simulink model "DynamicProprioTest"  (R2015a)
settings: Solver=ode4  SolverMode=MultiTasking  StartTime=0.0  StopTime=inf  FixedStep=BKIN_STEP_TIME  RelTol=1e-3
StartFcn:
  |  warndlg('Dexterit-E models cannot run under simulation. Please compile your model and run it from within Dexterit-E.');set_param(bdroot,'SimulationCommand','stop')
model workspace (MAT data in the model file):
  col_x = 1
  col_y = 2
  RADIUS_VIS = 3
  COLOR_INIT = 4
  BKIN_STEP_TIME = 0.00025
  START_WAIT_TIME_COL = 3
  E_END_TRIAL = 20
  STROKE_WIDTH = 6
  K_HAND_VEL = 1
  K_HOLDTIME = 2
  K_ROBOT_RAMP_TIME = 3
  E_ENABLED_CONTROLLER = 31
  K_TIME_TO_START = 4
  BKIN_KINEMATIC_FRAME_SIZE = 400
  E_NO_EVENT = 0
  ROTATION = 7
  E_WAIT_JS_THRESH = 16
  E_AT_JS_THRESH = 18
  STARTTARGET_COL = 1
  TIME_RETURNTOSTART_COL = 2
  MOVE_TIME_COL = 4
  TARGET_SHIFTTIME_COL = 5
  SHOWTARGETDUR_COL = 7
  MOVE_XVEL_COL = 9
  MOVE_YVEL_COL = 10
  E_INIT_TRIAL = 1
  E_MOVE_TO_START = 2
  E_AT_START = 4
  E_PASSIVE_HOLD_AT_START = 6
  E_MOVE_TO_END = 8
  COLOR_SELECT = 5
  ACTORPAS_COL = 11
  E_AT_END = 10
  DELAY_POSTTRIAL_COL = 8
  TARGETSHIFTDIR_COL = 6
  LABEL_HEIGHT = 8
  LABEL = 9
  E_ACTIVE_HOLD_AT_START = 7
  MVMT_VTHRESH_LB = 12
  MVMT_VTHRESH_UB = 13
  CHANNEL_WIDTH = 1
  WALL_WIDTH = 2
  WALL_STIFFNESS = 3
  WALL_VISCOSITY = 4
undefined symbols (not defined in the file): slselsubs
libraries: Video x6, simulink x5, slrtlib x5, General x3, KINARM_loads x3, KINARM_general x2, KINARM_IO x1, xpcnilib x1
(part 1 of 2)
CloseFcn:
  | rtwprivate ssgencode ModelCloseRequest b2lab2d
settings Model: ModifiedComment=chris -- Wed Feb 16 09:18:30 2005 -- Version 1.1384  ModifiedHistory=Feb 16/05 - Add error repeat, add offset ramp  ExtModeArmWhenConnect=off  ExtModeLogAll=off  Creator=Chris Grebeldinger  LastModifiedBy=User
settings SolverCC: EnableConcurrentExecution=on  AutoInsertRateTranBlk=on
settings DataIOCC: LimitDataPoints=off  SignalLoggingSaveFormat=ModelDataLogs  SaveOutput=off  SaveTime=off  SignalLoggingName=sigsOut
settings OptimizationCC: BlockReduction=off  BooleanDataType=off  OptimizeBlockIOStorage=off  BufferReuse=off  GlobalBufferReuse=off  ExpressionFolding=off  ExpressionDepthLimit=2147483647  LocalBlockOutputs=off  InitFltsAndDblsToZero=on
settings DebuggingCC: SaveWithParameterizedLinksMsg=none  UnderspecifiedInitializationDetection=Classic  MergeDetectMultiDrivingBlocksExec=none  SignalResolutionControl=TryResolveAllWithWarning  MultiTaskDSMMsg=warning  FcnCallInpInsideContextMsg=UseLocalSettings  StateNameClashWarn=warning  StrictBusMsg=ErrorOnBusTreatedAsVector
settings HardwareCC: ProdIntDivRoundTo=Zero  ProdEndianess=LittleEndian  ProdLongLongMode=on  ProdHWDeviceType=Generic->32-bit x86 compatible  TargetHWDeviceType=32-bit Generic
settings SFSimCC: SimCustomHeaderCode="#include \"stdlib.h\""  SFSimEcho=off  SimParseCustomCode=off
settings RTWCC: SystemTargetFile=slrt.tlc  TemplateMakefile=slrt_default_tmf  Description=Simulink Real-Time  CustomSourceCode="#include \"stdlib.h\""
settings CodeAppCC: MaxIdLength=63
settings SimulinkRealTimeCC: TargetFcnLib=ansi_tfl_tmw.mat  GeneratePreprocessorConditionals=Disable all  xPCisDownloadable=off  xPCisDefaultEnv=off

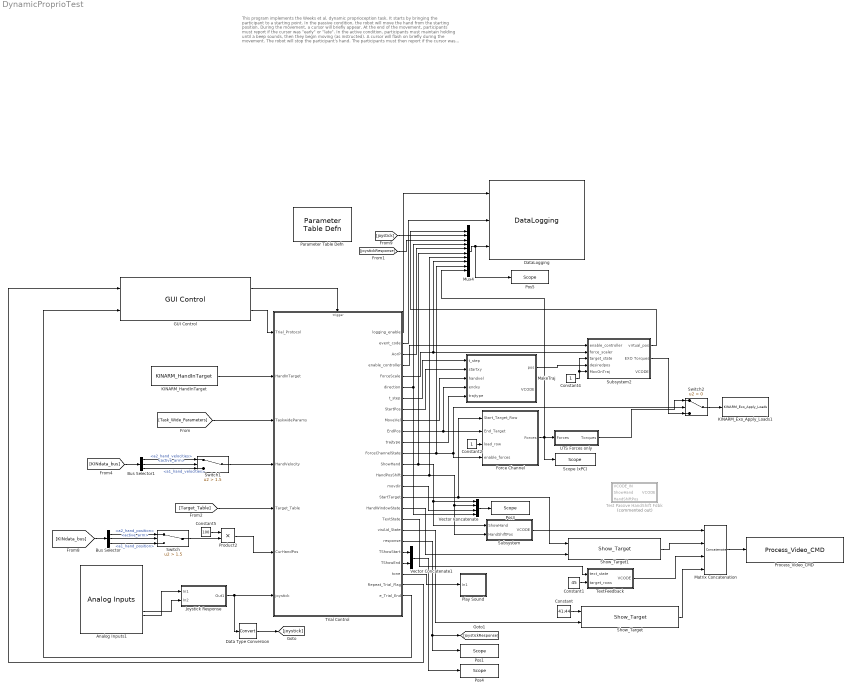
== system DynamicProprioTest ==
  note: This program implements the Weeks et al. dynamic proprioception task.
      | It starts by bringing the participant to a starting point.
      |
      | In the passive condition, the robot will move the hand from the starting position. During the movement, a cursor
      | will briefly appear. At the end of the movement, participants must report if the cursor was "early" or "late".
      |
      | In the active condition, participants must maintain holding
      | until a beep sounds, then they begin moving (as instructed). A cursor will flash on briefly during the movement.
      | The robot will stop the participant's hand. The participants must then report if the cursor was "early" or "late".
      | A force channel will enforce movement direction, and feedback will be used to adjust movement speed.
  Analog Inputs1 : KINARM_IO/Analog Inputs  channel=[1:32]  range=[5, 5, 5, 5, 5, 5, 5, 5,5, 5, 5, 5, 5, 5, 5, 5,5, 5, 5, 5, 5, 5, 5, 5,5, 5, 5, 5, 5, 5, 5, 5,]  coupling=[0, 0, 0, 0, 0, 0, 0, 0,0, 0, 0, 0, 0, 0, 0, 0,0, 0, 0, 0, 0, 0, 0, 0,0, 0, 0, 0, 0, 0, 0, 0,]  scantime6071e=1.28e-5  scantime6229=5e-6  sampletime=0.001  slot=-1  oscantime6071e=0
  Bus Selector : BusSelector  OutputSignals=Robot2.a2_hand_position,KINDataGeneral.active_arm,Robot1.a1_hand_position
  Bus Selector1 : BusSelector  OutputSignals=Robot2.a2_hand_velocities,KINDataGeneral.active_arm,Robot1.a1_hand_velocities
  Constant : Constant  Value=41:44
  Constant1 : Constant  Value=45
  Constant2 : Constant
  Constant4 : Constant
  Constant5 : Constant  Value=100
  Data Type Conversion : DataTypeConversion
  DataLogging : General/DataLogging  log_event_codes=on  log_analog_inputs=on  show_time_remaining=off
  Force Channel : Subsystem
  GUI Control : General/GUI Control  target_type_str=Circle  Target_Type=1  XYcols=[1 2]  Vcols=3  Lcols=4  indices_padding=[0 0 0 0;0 0 0 0]  task_version=1.0  show_repeat_trial_flag=on  target_table_rows=64  load_table_rows=20  tp_table_rows=100
  Joystick Response : Subsystem
  KINARM_Exo_Apply_Loads1 : KINARM_loads/KINARM_Exo_Apply_Loads  up_duration=200  down_duration=200  max_torque=12  limit_motors=off
  KINARM_HandInTarget : KINARM_general/KINARM_HandInTarget  use_dominant_hand=on  target_type=Rectangle  num_states=1  attribcol1=[RADIUS_VIS RADIUS_VIS 0]  attribcol2=[4 0 0]  attribcol3=[5 0 0]  attribcol4=[6 0 0]  attribcol5=[0 0 0]
  MakeTraj : Subsystem
  Matrix Concatenation : Concatenate  NumInputs=4  Mode=Multidimensional array
  Mux4 : Mux  Inputs=10
  Parameter Table Defn : General/Parameter Table Defn  ShowInLibBrowser=0
  Play Sound : Subsystem
  Pos1 : slrtlib/Displays and Logging/Scope   scopeno=2  scopetype=Target  autostart=on  viewmode=Numerical  formatstr='%15.6f'  grid=on  ylimits=[-10,10]  nosamples=250  noprepostsamples=0  interleave=1  triggermode=FreeRun  triggersignal=1  trigsignalfromport=off  triggerlevel=0.0  triggerslope=Either  triggerscope=1  triggersample=0  filename=data.dat  mode=Lazy  writesize=512  autorestart=off  dynamicfilemode=off  maxwritefilesize=512*1024^2
  Pos3 : slrtlib/Displays and Logging/Scope   scopeno=4  scopetype=Target  autostart=on  viewmode=Numerical  formatstr='%15.6f'  grid=on  ylimits=[-10,10]  nosamples=250  noprepostsamples=0  interleave=1  triggermode=FreeRun  triggersignal=1  trigsignalfromport=off  triggerlevel=0.0  triggerslope=Either  triggerscope=1  triggersample=0  filename=data.dat  mode=Lazy  writesize=512  autorestart=off  dynamicfilemode=off  maxwritefilesize=512*1024^2
  Pos4 : slrtlib/Displays and Logging/Scope   scopeno=5  scopetype=Target  autostart=on  viewmode=Numerical  formatstr='%15.6f'  grid=on  ylimits=[-10,10]  nosamples=250  noprepostsamples=0  interleave=1  triggermode=FreeRun  triggersignal=1  trigsignalfromport=off  triggerlevel=0.0  triggerslope=Either  triggerscope=1  triggersample=0  filename=data.dat  mode=Lazy  writesize=512  autorestart=off  dynamicfilemode=off  maxwritefilesize=512*1024^2
  Pos5 : slrtlib/Displays and Logging/Scope   scopeno=1  scopetype=Target  autostart=on  viewmode=Numerical  formatstr='%15.6f'  grid=on  ylimits=[-10,10]  nosamples=250  noprepostsamples=0  interleave=1  triggermode=FreeRun  triggersignal=1  trigsignalfromport=off  triggerlevel=0.0  triggerslope=Either  triggerscope=1  triggersample=0  filename=data.dat  mode=Lazy  writesize=512  autorestart=off  dynamicfilemode=off  maxwritefilesize=512*1024^2
  Process_Video_CMD : Video/Process_Video_CMD  video_delay=50
  Product2 : Product
  "Scope (xPC) " : slrtlib/Displays and Logging/Scope   scopeno=6  scopetype=Target  autostart=on  viewmode=Numerical  formatstr='%15.6f'  grid=on  ylimits=[0,0]  nosamples=250  noprepostsamples=0  interleave=1  triggermode=FreeRun  triggersignal=1  trigsignalfromport=off  triggerlevel=0.0  triggerslope=Either  triggerscope=1  triggersample=0  filename=data.dat  mode=Lazy  writesize=512  autorestart=off  dynamicfilemode=off  maxwritefilesize=512*1024^2
  Show_Target : Video/Show_Target  target_type=Triangle  num_states=2  attribcol1=[COLOR_INIT 0 0 RADIUS_VIS 0 0 ROTATION]  attribcol2=[COLOR_SELECT 0 0 RADIUS_VIS 0 0 ROTATION]  attribcol3=[0 0 0 0 0 0 0]  attribcol4=[0 0 0 0 0 0 0]  attribcol5=[0 0 24 0 0 0 0]  stateindices_padding=[0 0 0 0;0 0 0 0;0 0 0 0;0 0 0 0;0 0 0 0]  source=dialog  opacity=100  target_display=Both subject and operator displays  num_col=7
  Show_Target1 : Video/Show_Target  target_type=Rectangle  num_states=1  attribcol1=[0 COLOR_INIT STROKE_WIDTH RADIUS_VIS RADIUS_VIS 0]  attribcol2=[0 COLOR_SELECT 0 RADIUS_VIS 0 0]  attribcol3=[0 0 0 0 0 0]  attribcol4=[0 0 0 0 0 0]  attribcol5=[0 0 24 0 0 0]  stateindices_padding=[0 0 0 0 0;0 0 0 0 0;0 0 0 0 0;0 0 0 0 0;0 0 0 0 0]  source=dialog  opacity=100  target_display=Both subject and operator displays  num_col=6
  Subsystem : Subsystem
  Subsystem2 : Subsystem
  Switch : Switch  Criteria=u2 > Threshold  Threshold=1.5
  Switch1 : Switch  Criteria=u2 > Threshold  Threshold=1.5
  Switch2 : Switch  Criteria=u2 > Threshold
  Test Passive HandShift Fdbk : Subsystem  Commented=on
  TextFeedback : Subsystem
  Trial Control : Stateflow chart  TreatAsAtomicUnit=on
  UTS Forces only : Subsystem
  Vector Concatenate : Concatenate  NumInputs=4
  Vector Concatenate1 : Concatenate
  wires:
  [Task_Wide_Parameters] -> Trial Control/3(TaskwideParams)
  Trial Control/2(event_code) -> DataLogging/2
  Switch1/1 -> Trial Control/4(HandVelocity)
  Bus Selector1/3 -> Switch1/3  "<a1_hand_velocities>"
  Bus Selector1/1 -> Switch1/1  "<a2_hand_velocities>"
  [KINdata_bus] -> Bus Selector1/1
  GUI Control/2 -> Trial Control/1(Trial_Protocol)
  Trial Control/7(t_step) -> MakeTraj/1(t_step)
  KINARM_HandInTarget/1 -> Trial Control/2(HandInTarget)
  Trial Control/23(tone) -> Play Sound/1(In1)
  [Target_Table] -> Trial Control/5(Target_Table)
  Trial Control/24(Repeat_Trial_Flag) -> GUI Control/1
  GUI Control/1 -> Trial Control/Trigger
  Mux4/1 -> Pos5/1, DataLogging/3
  Trial Control/1(logging_enable) -> DataLogging/1
  Subsystem2/2(EXO Torques) -> Switch2/3
  Trial Control/25(e_Trial_End) -> GUI Control/2
  MakeTraj/1(pos) -> Subsystem2/4(desiredpos)
  Subsystem2/1(virtual_pos) -> Mux4/1
  Constant4/1 -> Subsystem2/3(target_state), Subsystem2/5(MovOnTraj)
  Trial Control/4(enable_controller) -> Subsystem2/1(enable_controller)
  [KINdata_bus] -> Bus Selector/1
  Bus Selector/2 -> Switch/2  "<active_arm>"
  Bus Selector/1 -> Switch/1  "<a2_hand_position>"
  Bus Selector/3 -> Switch/3  "<a1_hand_position>"
  Switch/1 -> Product2/2
  Constant5/1 -> Product2/1
  Product2/1 -> Trial Control/6(CurHandPos)
  Trial Control/6(direction) -> Mux4/4, Vector Concatenate/4
  Joystick Response/1(Out1) -> Data Type Conversion/1, Trial Control/7(joystick)
  Matrix Concatenation/1 -> Process_Video_CMD/1
  Analog Inputs1/24 -> Joystick Response/1(In1)
  Analog Inputs1/22 -> Joystick Response/2(In2)
  Trial Control/20(response) -> [joystickResponse], Pos1/1
  [joystick] -> Mux4/2
  Data Type Conversion/1 -> [joystick]
  Trial Control/8(StartPos) -> MakeTraj/2(startxy)
  Trial Control/9(MoveVel) -> MakeTraj/3(handvel)
  Trial Control/10(EndPos) -> MakeTraj/4(endxy), Force Channel/2(End_Target)
  Trial Control/11(trajtype) -> MakeTraj/5(trajtype)
  Trial Control/13(ShowHand) -> Vector Concatenate/1, Subsystem/1(ShowHand), Mux4/6
  Subsystem/1(VCODE) -> Matrix Concatenation/1
  Trial Control/19(visAid_State) -> Show_Target/2
  Constant/1 -> Show_Target/1
  Show_Target/1 -> Matrix Concatenation/4
  Trial Control/3(AorP) -> Mux4/5
  Vector Concatenate/1 -> Pos3/1
  Trial Control/21(TShowStart) -> Vector Concatenate1/1
  Trial Control/22(TShowEnd) -> Vector Concatenate1/2
  Vector Concatenate1/1 -> Pos4/1
  Force Channel/1(Forces) -> "Scope (xPC) "/1, Mux4/10, UTS Forces only/1(Forces)
  UTS Forces only/1(Torques) -> Switch2/1
  Trial Control/15(movdir) -> Vector Concatenate/3
  Show_Target1/1 -> Matrix Concatenation/2
  Trial Control/17(HandWindowState) -> Show_Target1/2
  Trial Control/5(ForceScale) -> Subsystem2/2(force_scaler), Mux4/8
  TextFeedback/1(VCODE) -> Matrix Concatenation/3
  Constant1/1 -> TextFeedback/2(target_rows)
  Trial Control/18(TextState) -> TextFeedback/1(text_state)
  Bus Selector1/2 -> Switch1/2  "<active_arm>"
  Trial Control/16(StartTarget) -> Show_Target1/1, Force Channel/1(Start_Target_Row)
  Constant2/1 -> Force Channel/3(load_row)
  Trial Control/12(ForceChannelState) -> Switch2/2, Force Channel/4(enable_forces), Mux4/9
  Switch2/1 -> KINARM_Exo_Apply_Loads1/1
  Trial Control/14(HandPosShift) -> Mux4/7, Subsystem/2(HandShiftPos), Vector Concatenate/2
  [joystickResponse] -> Mux4/3

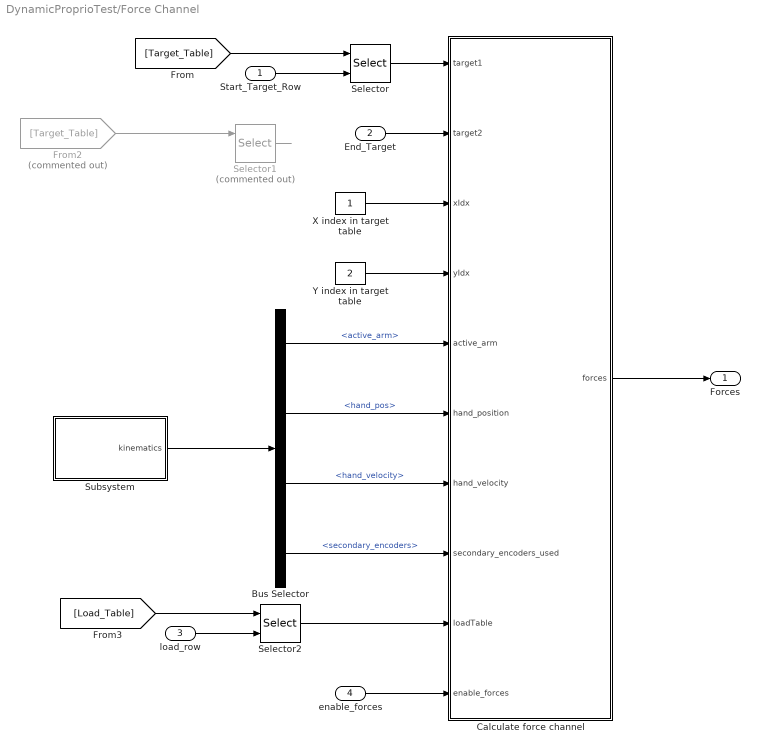
== system DynamicProprioTest/Force Channel ==
  Start_Target_Row : Inport
  End_Target : Inport  Port=2
  load_row : Inport  Port=3
  enable_forces : Inport  Port=4
  Bus Selector : BusSelector  OutputSignals=active_arm,hand_pos,hand_velocity,secondary_encoders
  Calculate force channel : MATLAB Function  TreatAsAtomicUnit=on
  From2 : From  Commented=on  GotoTag=Target_Table  TagVisibility=global
      settings: CloseFcn=tagdialog Close
  Selector : Selector  NumberOfDimensions=2  InputPortWidth=3  IndexOptions=Index vector (port),Select all  Indices=1,-1  OutputSizes=slselsubs([(-2),(-2)],1),slselsubs([(-2),(-2)],2)
  Selector1 : Selector  Commented=on  NumberOfDimensions=2  InputPortWidth=3  IndexOptions=Index vector (port),Select all  Indices=1,-1  OutputSizes=slselsubs([(-2),(-2)],1),slselsubs([(-2),(-2)],2)
  Selector2 : Selector  NumberOfDimensions=2  InputPortWidth=3  IndexOptions=Index vector (port),Select all  Indices=1,-1  OutputSizes=slselsubs([(-2),(-2)],1),slselsubs([(-2),(-2)],2)
  Subsystem : Subsystem
  X index in target table : Constant
  Y index in target table : Constant  Value=2
  Forces : Outport
  wires:
  Selector/1 -> Calculate force channel/1(target1)
  [Target_Table] -> Selector/1
  Start_Target_Row/1 -> Selector/2
  Selector1/1 -> ?
  From2/1 -> Selector1/1
  End_Target/1 -> Calculate force channel/2(target2)
  X index in target table/1 -> Calculate force channel/3(xIdx)
  Y index in target table/1 -> Calculate force channel/4(yIdx)
  enable_forces/1 -> Calculate force channel/10(enable_forces)
  [Load_Table] -> Selector2/1
  load_row/1 -> Selector2/2
  Selector2/1 -> Calculate force channel/9(loadTable)
  Calculate force channel/1(forces) -> Forces/1
  Subsystem/1(kinematics) -> Bus Selector/1
  Bus Selector/1 -> Calculate force channel/5(active_arm)  "<active_arm>"
  Bus Selector/2 -> Calculate force channel/6(hand_position)  "<hand_pos>"
  Bus Selector/3 -> Calculate force channel/7(hand_velocity)  "<hand_velocity>"
  Bus Selector/4 -> Calculate force channel/8(secondary_encoders_used)  "<secondary_encoders>"

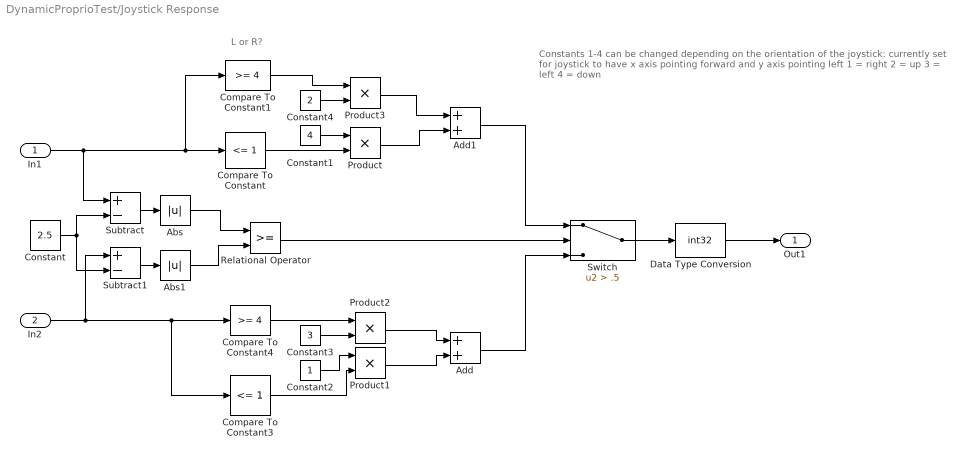
== system DynamicProprioTest/Joystick Response ==
  note: Constants 1-4 can be changed depending on the orientation of the joystick:
      | currently set for joystick to have x axis pointing forward and y axis pointing left
      |
      | 1 = right
      | 2 = up
      | 3 = left
      | 4 = down
  note: L or R?
  In1 : Inport
  In2 : Inport  Port=2
  Abs : Abs
  Abs1 : Abs
  Add : Sum
  Add1 : Sum
  Compare To Constant : simulink/Logic and Bit Operations/Compare To Constant  relop=<=  const=1  OutDataTypeStr=boolean
  Compare To Constant1 : simulink/Logic and Bit Operations/Compare To Constant  relop=>=  const=4  OutDataTypeStr=boolean
  Compare To Constant3 : simulink/Logic and Bit Operations/Compare To Constant  relop=<=  const=1  OutDataTypeStr=boolean
  Compare To Constant4 : simulink/Logic and Bit Operations/Compare To Constant  relop=>=  const=4  OutDataTypeStr=boolean
  Constant : Constant  Value=2.5
  Constant1 : Constant  Value=4
  Constant2 : Constant
  Constant3 : Constant  Value=3
  Constant4 : Constant  Value=2
  Data Type Conversion : DataTypeConversion  OutDataTypeStr=int32
  Product{,1..3} (4 alike) : Product
  Relational Operator : RelationalOperator  OutDataTypeStr=boolean
  Subtract : Sum  Inputs=+-
  Subtract1 : Sum  Inputs=+-
  Switch : Switch  Criteria=u2 > Threshold  Threshold=.5
  Out1 : Outport
  wires:
  In1/1 -> Subtract/1, Compare To Constant1/1, Compare To Constant/1
  Compare To Constant/1 -> Product/2
  In2/1 -> Subtract1/1, Compare To Constant3/1, Compare To Constant4/1
  Compare To Constant3/1 -> Product1/2
  Compare To Constant4/1 -> Product2/1
  Subtract/1 -> Abs/1
  Subtract1/1 -> Abs1/1
  Constant/1 -> Subtract/2, Subtract1/2
  Abs/1 -> Relational Operator/1
  Abs1/1 -> Relational Operator/2
  Compare To Constant1/1 -> Product3/1
  Constant1/1 -> Product/1
  Constant2/1 -> Product1/1
  Constant3/1 -> Product2/2
  Product2/1 -> Add/1
  Product1/1 -> Add/2
  Product/1 -> Add1/2
  Add1/1 -> Switch/1
  Add/1 -> Switch/3
  Relational Operator/1 -> Switch/2
  Constant4/1 -> Product3/2
  Product3/1 -> Add1/1
  Switch/1 -> Data Type Conversion/1
  Data Type Conversion/1 -> Out1/1

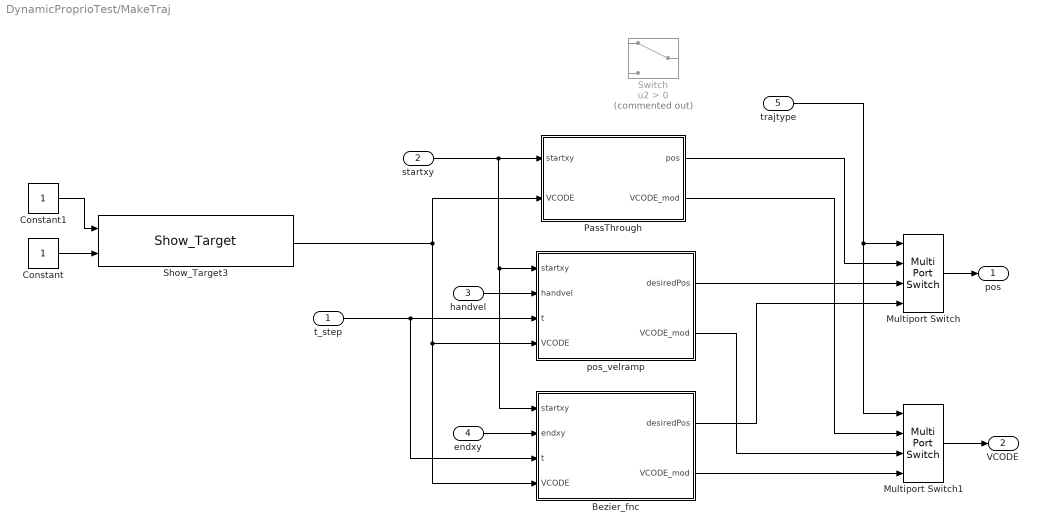
== system DynamicProprioTest/MakeTraj ==
  t_step : Inport  PortDimensions=1
  startxy : Inport  Port=2  PortDimensions=[1 2]
  handvel : Inport  Port=3
  endxy : Inport  Port=4
  trajtype : Inport  Port=5  PortDimensions=1
  Bezier_fnc : MATLAB Function  TreatAsAtomicUnit=on
  Constant : Constant
  Constant1 : Constant
  Multiport Switch : MultiPortSwitch  DataPortOrder=Specify indices  DataPortIndices={2,1,0}  DiagnosticForDefault=Warning
  Multiport Switch1 : MultiPortSwitch  DataPortOrder=Specify indices  DataPortIndices={2,1,0}  DiagnosticForDefault=Warning
  PassThrough : MATLAB Function  TreatAsAtomicUnit=on
  Show_Target3 : Video/Show_Target  target_type=Circle  num_states=1  attribcol1=[COLOR_INIT 0 0 RADIUS_VIS]  attribcol2=[6 6 0 3]  attribcol3=[0 0 0 0]  attribcol4=[0 0 0 0]  attribcol5=[0 0 24 0]  stateindices_padding=[0 0 0 0 0 0 0;0 0 0 0 0 0 0;0 0 0 0 0 0 0;0 0 0 0 0 0 0;0 0 0 0 0 0 0]  source=dialog  opacity=100  target_display=Both subject and operator displays  num_col=4
  Switch : Switch  Commented=on  Criteria=u2 > Threshold
  pos_velramp : MATLAB Function  TreatAsAtomicUnit=on
  pos : Outport  OutDataTypeStr=double  PortDimensions=[1 2]
  VCODE : Outport  Port=2
  wires:
  Show_Target3/1 -> Bezier_fnc/4(VCODE), pos_velramp/4(VCODE), PassThrough/2(VCODE)
  Constant1/1 -> Show_Target3/1
  startxy/1 -> Bezier_fnc/1(startxy), pos_velramp/1(startxy), PassThrough/1(startxy)
  Constant/1 -> Show_Target3/2
  t_step/1 -> Bezier_fnc/3(t), pos_velramp/3(t)
  handvel/1 -> pos_velramp/2(handvel)
  endxy/1 -> Bezier_fnc/2(endxy)
  Multiport Switch/1 -> pos/1
  Multiport Switch1/1 -> VCODE/1
  pos_velramp/1(desiredPos) -> Multiport Switch/3
  Bezier_fnc/1(desiredPos) -> Multiport Switch/4
  pos_velramp/2(VCODE_mod) -> Multiport Switch1/3
  Bezier_fnc/2(VCODE_mod) -> Multiport Switch1/4
  trajtype/1 -> Multiport Switch1/1, Multiport Switch/1
  PassThrough/1(pos) -> Multiport Switch/2
  PassThrough/2(VCODE_mod) -> Multiport Switch1/2

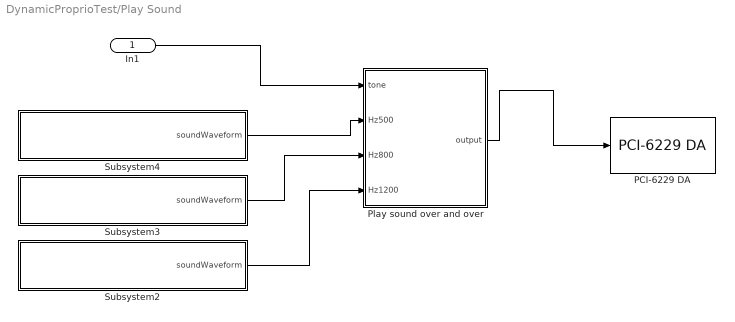
== system DynamicProprioTest/Play Sound ==
  In1 : Inport
  PCI-6229 DA : xpcnilib/D//A/M Series/PCI-6229 DA  channel=[1]  reset=[1]  initValue=[0]  sampletime=-1  slot=-1
  Play sound over and over : MATLAB Function  TreatAsAtomicUnit=on
  Subsystem2 : Subsystem  mask(Load Waveform Into Variable){fileName=Hz1200}
      mask prompts: fileName "Name of .mat Data File (must be in current directory)"
      mask help: This block will load the .MAT file specified in the dialog, and put the first variable into a GoTo called 'soundWaveform'.
      mask init:
      | filenameFromMask = get_param(gcb, 'fileName');
      | 
      | try 
      | 	dataFromFile = load(filenameFromMask);
      | 	names = fieldnames(dataFromFile);
      | 	soundDataFromFile = dataFromFile.(names{1});
      | 	display(['Sound waveform from file ''' filenameFromMask ''' loaded.']);
      | catch ME
      | 	display(ME.message)
      | end
      mask Help:
      | Enter the name a .MAT file containing a single vector or matrix. The .MAT file must be located in the current directory.
      | 
      | The first variable from the .MAT file will be put into a Goto called 'soundWaveform'.
      mask Display: disp(['Load waveform from ''' filenameFromMask ''''])
  Subsystem3 : Subsystem  mask(Load Waveform Into Variable){fileName=Hz800}
      mask prompts: fileName "Name of .mat Data File (must be in current directory)"
      mask help: This block will load the .MAT file specified in the dialog, and put the first variable into a GoTo called 'soundWaveform'.
      mask init: same as DynamicProprioTest/Play Sound/Subsystem2
      mask Help:
      | Enter the name a .MAT file containing a single vector or matrix. The .MAT file must be located in the current directory.
      | 
      | The first variable from the .MAT file will be put into a Goto called 'soundWaveform'.
      mask Display: disp(['Load waveform from ''' filenameFromMask ''''])
  Subsystem4 : Subsystem  mask(Load Waveform Into Variable){fileName=Hz500}
      mask prompts: fileName "Name of .mat Data File (must be in current directory)"
      mask help: This block will load the .MAT file specified in the dialog, and put the first variable into a GoTo called 'soundWaveform'.
      mask init: same as DynamicProprioTest/Play Sound/Subsystem2
      mask Help:
      | Enter the name a .MAT file containing a single vector or matrix. The .MAT file must be located in the current directory.
      | 
      | The first variable from the .MAT file will be put into a Goto called 'soundWaveform'.
      mask Display: disp(['Load waveform from ''' filenameFromMask ''''])
  wires:
  Play sound over and over/1(output) -> PCI-6229 DA/1
  Subsystem3/1(soundWaveform) -> Play sound over and over/3(Hz800)
  Subsystem4/1(soundWaveform) -> Play sound over and over/2(Hz500)
  In1/1 -> Play sound over and over/1(tone)
  Subsystem2/1(soundWaveform) -> Play sound over and over/4(Hz1200)

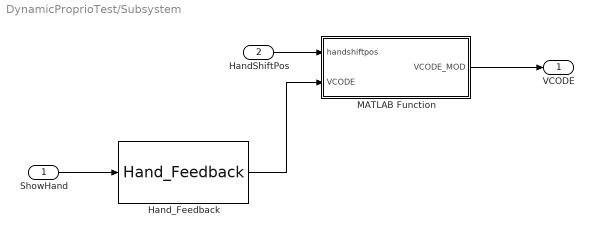
== system DynamicProprioTest/Subsystem ==
  ShowHand : Inport
  HandShiftPos : Inport  Port=2
  Hand_Feedback : KINARM_general/Hand_Feedback  feedback_cntl_src=status only
  MATLAB Function : MATLAB Function  TreatAsAtomicUnit=on
  VCODE : Outport
  wires:
  ShowHand/1 -> Hand_Feedback/1
  HandShiftPos/1 -> MATLAB Function/1(handshiftpos)
  Hand_Feedback/1 -> MATLAB Function/2(VCODE)
  MATLAB Function/1(VCODE_MOD) -> VCODE/1

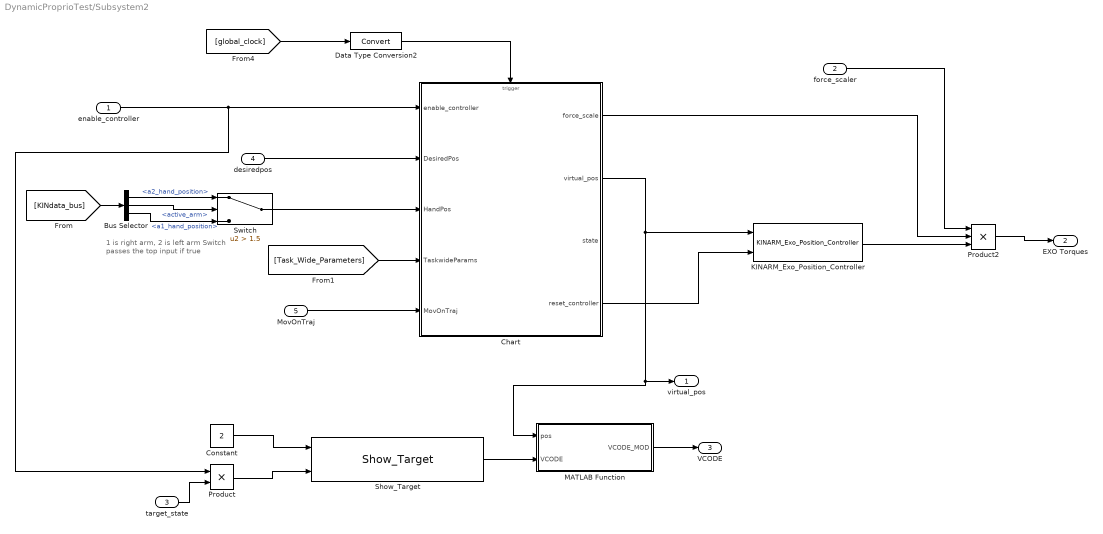
== system DynamicProprioTest/Subsystem2 ==
  note: 1 is right arm, 2 is left arm
      | Switch passes the top input if true
  enable_controller : Inport
  force_scaler : Inport  Port=2
  target_state : Inport  Port=3
  desiredpos : Inport  Port=4
  MovOnTraj : Inport  Port=5
  Bus Selector : BusSelector  OutputSignals=Robot2.a2_hand_position,KINDataGeneral.active_arm,Robot1.a1_hand_position
  Chart : Stateflow chart  TreatAsAtomicUnit=on
  Constant : Constant  Value=2
  Data Type Conversion2 : DataTypeConversion
  KINARM_Exo_Position_Controller : KINARM_loads/KINARM_Exo_Position_Controller  use_dom_hand=on  KINARM_Type=Human  inertias_for_FF=KINARM robot & arm troughs & subject  angles_or_XY=End-point (global x/y)  sample_time=0.001
  MATLAB Function : MATLAB Function  TreatAsAtomicUnit=on
  Product : Product
  Product2 : Product  Inputs=3
  Show_Target : Video/Show_Target  target_type=Circle  num_states=1  attribcol1=[COLOR_INIT 0 0 RADIUS_VIS]  attribcol2=[6 6 0 3]  attribcol3=[0 0 0 0]  attribcol4=[0 0 0 0]  attribcol5=[0 0 24 0]  stateindices_padding=[0 0 0 0 0 0 0;0 0 0 0 0 0 0;0 0 0 0 0 0 0;0 0 0 0 0 0 0;0 0 0 0 0 0 0]  source=dialog  opacity=100  target_display=Both subject and operator displays  num_col=4
  Switch : Switch  Criteria=u2 > Threshold  Threshold=1.5
  virtual_pos : Outport
  EXO Torques : Outport  Port=2
  VCODE : Outport  Port=3
  wires:
  [KINdata_bus] -> Bus Selector/1
  Bus Selector/2 -> Switch/2  "<active_arm>"
  [Task_Wide_Parameters] -> Chart/4(TaskwideParams)
  [global_clock] -> Data Type Conversion2/1
  Data Type Conversion2/1 -> Chart/Trigger
  Chart/2(virtual_pos) -> MATLAB Function/1(pos), virtual_pos/1, KINARM_Exo_Position_Controller/1
  MovOnTraj/1 -> Chart/5(MovOnTraj)
  Switch/1 -> Chart/3(HandPos)
  desiredpos/1 -> Chart/2(DesiredPos)
  Constant/1 -> Show_Target/1
  Show_Target/1 -> MATLAB Function/2(VCODE)
  MATLAB Function/1(VCODE_MOD) -> VCODE/1
  KINARM_Exo_Position_Controller/1 -> Product2/3
  Product2/1 -> EXO Torques/1
  Chart/1(force_scale) -> Product2/2
  Chart/4(reset_controller) -> KINARM_Exo_Position_Controller/2
  Bus Selector/1 -> Switch/1  "<a2_hand_position>"
  Bus Selector/3 -> Switch/3  "<a1_hand_position>"
  enable_controller/1 -> Product/1, Chart/1(enable_controller)
  Product/1 -> Show_Target/2
  target_state/1 -> Product/2
  force_scaler/1 -> Product2/1

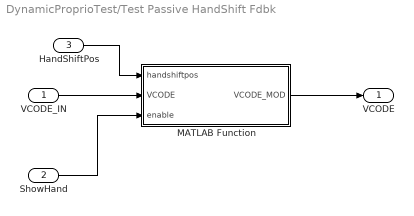
== system DynamicProprioTest/Test Passive HandShift Fdbk ==
  VCODE_IN : Inport
  ShowHand : Inport  Port=2
  HandShiftPos : Inport  Port=3
  MATLAB Function : MATLAB Function  TreatAsAtomicUnit=on
  VCODE : Outport
  wires:
  HandShiftPos/1 -> MATLAB Function/1(handshiftpos)
  MATLAB Function/1(VCODE_MOD) -> VCODE/1
  VCODE_IN/1 -> MATLAB Function/2(VCODE)
  ShowHand/1 -> MATLAB Function/3(enable)

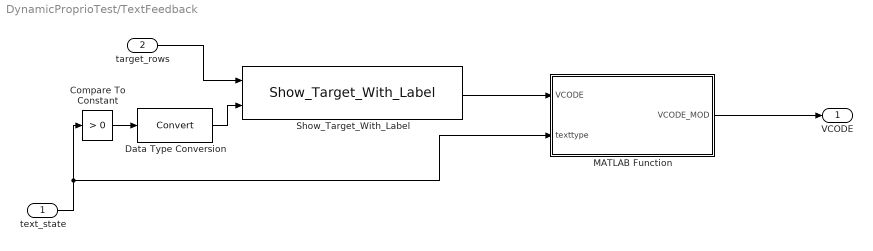
== system DynamicProprioTest/TextFeedback ==
  text_state : Inport
  target_rows : Inport  Port=2
  Compare To Constant : simulink/Logic and Bit Operations/Compare To Constant  relop=>  const=0  OutDataTypeStr=boolean
  Data Type Conversion : DataTypeConversion
  MATLAB Function : MATLAB Function  TreatAsAtomicUnit=on
  Show_Target_With_Label : Video/Show_Target_With_Label  target_type=Circle  num_states=1  attribcol1=[0 0 0 RADIUS_VIS LABEL COLOR_INIT LABEL_HEIGHT]  attribcol2=[6 6 0 3 0 0 0]  attribcol3=[0 0 0 0 0 0 0]  attribcol4=[0 0 0 0 0 0 0]  attribcol5=[0 0 24 0 0 0 0]  stateindices_padding=[0 0 0 0;0 0 0 0;0 0 0 0;0 0 0 0;0 0 0 0]  source=dialog  opacity=100  target_display=Both subject and operator displays
  VCODE : Outport
  wires:
  target_rows/1 -> Show_Target_With_Label/1
  text_state/1 -> MATLAB Function/2(texttype), Compare To Constant/1
  Show_Target_With_Label/1 -> MATLAB Function/1(VCODE)
  MATLAB Function/1(VCODE_MOD) -> VCODE/1
  Compare To Constant/1 -> Data Type Conversion/1
  Data Type Conversion/1 -> Show_Target_With_Label/2

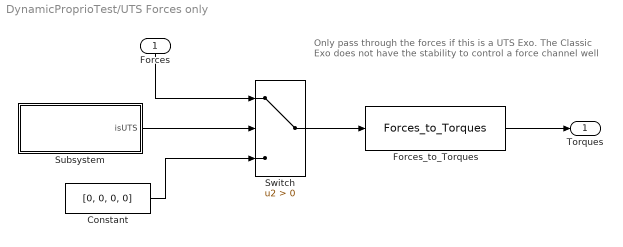
== system DynamicProprioTest/UTS Forces only ==
  note: Only pass through the forces if this is a UTS Exo. The
      | Classic Exo does not have the stability to control a
      | force channel well
  Forces : Inport
  Constant : Constant  Value=[0, 0, 0, 0]
  Forces_to_Torques : KINARM_loads/Forces_to_Torques
  Subsystem : Subsystem
  Switch : Switch  Criteria=u2 > Threshold
  Torques : Outport
  wires:
  Subsystem/1(isUTS) -> Switch/2
  Constant/1 -> Switch/3
  Switch/1 -> Forces_to_Torques/1
  Forces/1 -> Switch/1
  Forces_to_Torques/1 -> Torques/1

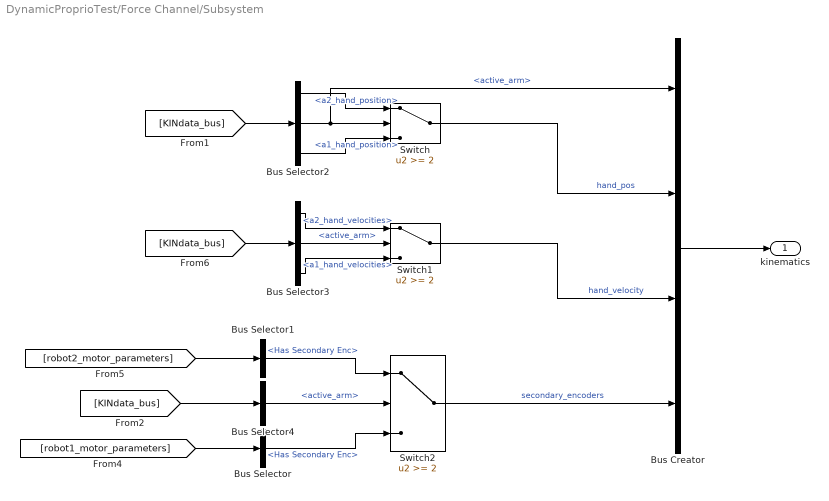
== system DynamicProprioTest/Force Channel/Subsystem ==
  Bus Creator : BusCreator
  Bus Selector : BusSelector  OutputSignals=R1.Has Secondary Enc
  Bus Selector1 : BusSelector  OutputSignals=R2.Has Secondary Enc
  Bus Selector2 : BusSelector  OutputSignals=Robot2.a2_hand_position,KINDataGeneral.active_arm,Robot1.a1_hand_position
  Bus Selector3 : BusSelector  OutputSignals=Robot2.a2_hand_velocities,KINDataGeneral.active_arm,Robot1.a1_hand_velocities
  Bus Selector4 : BusSelector  OutputSignals=KINDataGeneral.active_arm
  Switch : Switch  Threshold=2
  Switch1 : Switch  Threshold=2
  Switch2 : Switch  Threshold=2
  kinematics : Outport
  wires:
  [KINdata_bus] -> Bus Selector2/1
  Bus Selector2/1 -> Switch/1  "<a2_hand_position>"
  Bus Selector2/3 -> Switch/3  "<a1_hand_position>"
  Bus Selector2/2 -> Bus Creator/1, Switch/2  "<active_arm>"
  Bus Selector3/1 -> Switch1/1  "<a2_hand_velocities>"
  Bus Selector3/2 -> Switch1/2  "<active_arm>"
  Bus Selector3/3 -> Switch1/3  "<a1_hand_velocities>"
  [KINdata_bus] -> Bus Selector3/1
  [robot2_motor_parameters] -> Bus Selector1/1
  [robot1_motor_parameters] -> Bus Selector/1
  Bus Selector/1 -> Switch2/3  "<Has Secondary Enc>"
  Bus Selector1/1 -> Switch2/1  "<Has Secondary Enc>"
  [KINdata_bus] -> Bus Selector4/1
  Bus Selector4/1 -> Switch2/2  "<active_arm>"
  Switch/1 -> Bus Creator/2  "hand_pos"
  Switch1/1 -> Bus Creator/3  "hand_velocity"
  Switch2/1 -> Bus Creator/4  "secondary_encoders"
  Bus Creator/1 -> kinematics/1

== system DynamicProprioTest/Play Sound/Subsystem2 ==
  Constant1 : Constant  Value=soundDataFromFile  SampleTime=-1
  soundWaveform : Outport
  wires:
  Constant1/1 -> soundWaveform/1

== system DynamicProprioTest/Play Sound/Subsystem3 ==
  Constant1 : Constant  Value=soundDataFromFile
  soundWaveform : Outport
  wires:
  Constant1/1 -> soundWaveform/1

== system DynamicProprioTest/Play Sound/Subsystem4 ==
  Constant1 : Constant  Value=soundDataFromFile
  soundWaveform : Outport
  wires:
  Constant1/1 -> soundWaveform/1

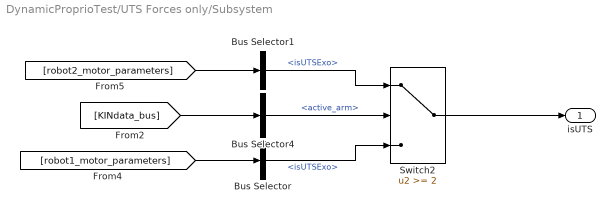
== system DynamicProprioTest/UTS Forces only/Subsystem ==
  Bus Selector : BusSelector  OutputSignals=R1Info.isUTSExo
  Bus Selector1 : BusSelector  OutputSignals=R2Info.isUTSExo
  Bus Selector4 : BusSelector  OutputSignals=KINDataGeneral.active_arm
  Switch2 : Switch  Threshold=2
  isUTS : Outport
  wires:
  [robot1_motor_parameters] -> Bus Selector/1
  Bus Selector4/1 -> Switch2/2  "<active_arm>"
  Switch2/1 -> isUTS/1
  Bus Selector1/1 -> Switch2/1  "<isUTSExo>"
  [KINdata_bus] -> Bus Selector4/1
  [robot2_motor_parameters] -> Bus Selector1/1
  Bus Selector/1 -> Switch2/3  "<isUTSExo>"

== matlab function DynamicProprioTest/MakeTraj/Bezier_fnc ==
  data: startxy input size=[1 2]; endxy input; t input; desiredPos output size=[1 2]; VCODE input; VCODE_mod output
function [desiredPos,VCODE_mod] = fcn(startxy,endxy,t,VCODE)
%#codegen

VCODE_mod = VCODE;

%clip t just in case!
if t < 0
    t = 0;
elseif t > 1;
    t = 1;
end

t = t-sin(2*pi*t)/(2*pi);  %use the bell-shaped velocity profile from the trajectory controller

%linear bezier using origin and reference
%point from the next trial
cp1 = startxy;
cp2 = endxy;

dPos = (1-t)*cp1 + t*cp2;


desiredPos = dPos; %to get to cm
desiredPos = desiredPos/100;

VCODE_mod(3) = desiredPos(1); %convert to meters
VCODE_mod(4) = desiredPos(2); %convert to meters

== matlab function DynamicProprioTest/Subsystem/MATLAB Function ==
  data: handshiftpos input; VCODE_MOD output; VCODE input
function VCODE_MOD = fcn(handshiftpos,VCODE)
%#codegen

%already in meters
%handshiftpos = handshiftpos/100;



VCODE(1,3)=VCODE(1,3)+handshiftpos(1);          %target position in m
VCODE(1,4)=VCODE(1,4)+handshiftpos(2);			%target position in m


VCODE_MOD = VCODE;

== matlab function DynamicProprioTest/Test Passive HandShift Fdbk/MATLAB Function ==
  data: handshiftpos input; VCODE_MOD output; VCODE input; enable input
function VCODE_MOD = fcn(handshiftpos,VCODE,enable)
%#codegen

%already in m
%handshiftpos = handshiftpos/100;


if (enable == 0)
    VCODE(:,2) = 0;
else
    VCODE(:,2) = 1;
end


VCODE(1,3)=VCODE(1,3)+handshiftpos(1);          %target position in m
VCODE(1,4)=VCODE(1,4)+handshiftpos(2);			%target position in m


VCODE_MOD = VCODE;

== matlab function DynamicProprioTest/Play Sound/Play sound over and over ==
  data: tone input; output output; Hz500 input; Hz800 input; Hz1200 input
function output = fcn(tone,Hz500,Hz800,Hz1200)
%#codegen

persistent t last_tone_state
if isempty(t), t = 0; end
if isempty(last_tone_state), last_tone_state = 0; end

trigger = last_tone_state ~= tone;
if trigger > 0
    last_tone_state = tone;
end

output = 0;		% default
if t == 0 && trigger > 0
	% start the playing of the sound.
	t = t + 1;
end

if tone == 1
    data = Hz500;
elseif tone == 2
    data = Hz800;
elseif tone == 3
    data = Hz1200;
else 
    t = 0;
    data = 0;
end

if t > 0
	output = data(t);
	if t == length(data)
		t = 0;
	else
		t = t + 1;
	end
end

== matlab function DynamicProprioTest/Force Channel/Calculate force channel ==
  data: target1 input; forces output; target2 input; xIdx input; yIdx input; active_arm input; hand_position input; hand_velocity input; secondary_encoders_used input; loadTable input; enable_forces input
function forces = forceChannel(target1, target2, xIdx, yIdx, active_arm, hand_position, hand_velocity, secondary_encoders_used, loadTable, enable_forces)

	persistent lastForcesEnabledValue forceEnableTime clockCycle outsideChannel lastHandPosition;
	
	if isempty(lastForcesEnabledValue), lastForcesEnabledValue = 0;		end
	if isempty(forceEnableTime),        forceEnableTime = 1;			end
	if isempty(clockCycle),				clockCycle = 0;					end
	if isempty(outsideChannel),			outsideChannel = 0;				end
	if isempty(lastHandPosition),		lastHandPosition = zeros(1,2);	end


	%we need to keep track of the time so we can safely ramp up forces when 
	%the trial starts.
	clockCycle = clockCycle + 1;
	if lastForcesEnabledValue == 0 && enable_forces == 1
		forceEnableTime = clockCycle;
	end

	lastForcesEnabledValue = enable_forces;

	%start out assuming we will apply no forces.
	forces = zeros(1, 4);

    channelWidthM = abs((loadTable(1) * 0.01) / 2.0);%get the width of the zero force zone and convert to meters
	wallWidthM = abs(loadTable(2) * 0.01);			%get the width of the wall where forces cut out and convert to meters.
%     if secondary_encoders_used == 0
%         % No secondary encoders
%     	wallStiffness = abs(loadTable(3));				%in N/m
%     	viscosity = -abs(loadTable(4));					%in N/(m/s)
%     else
        % With secondary encoders
    	wallStiffness = abs(loadTable(3));				%in N/m
    	viscosity = -abs(loadTable(4));					%in N/(m/s)
%     end

	xHand=hand_position(1);		%(m)
	yHand=hand_position(2);		%(m)

	%get the target positions and convert them to meters.
	x1 = target1(xIdx) * 0.01;
	y1 = target1(yIdx) * 0.01;
	x2 = target2(1) * 0.01;  %target 2 is projected from target1 and the desired start velocities
	y2 = target2(2) * 0.01;

	%http://www.codeguru.com/forum/showthread.php?threadid=194400
	%This calculations gives us the distance away from the line we are now.
	distToLine = abs(((x2 - x1)*(y1-yHand)) - ((x1 - xHand)*(y2-y1))) / sqrt( (x2 - x1)^2 + (y2 - y1)^2 );

	HXVEL = hand_velocity(1);
	HYVEL = hand_velocity(2);
	viscosityX = HXVEL * viscosity;
	viscosityY = HYVEL * viscosity;

	%we only ever want to provide a viscous load perpendicular to
	%the force channel. This viscous force will be used to dampen
	%any instability.
	if (x2 == x1) %infinite slope
		viscosityY = 0;	
	elseif (y2 == y1) %0 slope
		viscosityX = 0;
	else
		m = (y2 - y1) / (x2 - x1);
		perpM = -(1/m);	

		%we need to scale the viscous load to only the components
		%that are perpendicular to the line. To do that we find the 
		%projection of the velocity vecotor on a line perpendicular to the
		%force channel
		perpVect = [1 perpM];
		perpUnitVector = perpVect / norm(perpVect);

		%this finds the projection of the vector perpendicular to the channel
		dotProduct = dot([viscosityX viscosityY], perpUnitVector);
		scaledForces = dotProduct * perpUnitVector;

		viscosityX = scaledForces(1);
		viscosityY = scaledForces(2);
	end

	%forces 1,2 are for right arm, 3,4 are for left
	addIdx = 0;
	if active_arm == 2
		addIdx = 2;
	end

	% if we are outside the force wall we need to make sure we don't turn it
	%back on until we are in the channel. Otherwise it's quite jarring to be pulled in.
	if distToLine > (wallWidthM + channelWidthM)
		outsideChannel = 1;
		return
	elseif enable_forces == 0
		return	
	%if we are in the force channel we still need to viscous loads to aid in stability
	%if we are bouncing between the walls. 
	elseif distToLine < channelWidthM 
		outsideChannel = 0; %we're in the channel, so we can turn forces back on if they were off.
		return
	elseif outsideChannel == 1    
		%If we were outside the wall then forces are all off. We only want to turn
		%forces back on if the hand has crossed the line of the force channel, that way
		%you are not pushed into the channel, it only feels like you hit a wall.
		%By looking at the previous hand position and the current hand position
		%we can see if that line segment crosses the channel line, in which case we can
		%turn the forces back on.
		if doLinesIntersect([x1 y1], [x2 y2], [xHand yHand], lastHandPosition) == 1
			outsideChannel = 0;
		else
			return
		end
	end

	distIntoWall = distToLine - channelWidthM;

	if (x2 == x1) %all force wille be in x direction
		y = 0;
		if xHand < x1
			x = distIntoWall;
		else
			x = -distIntoWall;
		end
	elseif (y2 == y1) %all force will be in Y direction
		x = 0;
		if yHand < y1
			y = distIntoWall;
		else
			y = -distIntoWall;
		end	
	else
		%we need to find out how far off the line in X and Y we are in meters so 
		%we can properly convert the wall stiffness in N/m to a force.
		m = (y2 - y1) / (x2 - x1);
		b = y1 - (m * x1);

		perpM = -(1/m);	
		perpB = yHand - (perpM * xHand);

		xIntersect = (b - perpB) / (perpM - m);
		yIntersect = (m * xIntersect) + b;

		%x and y are converted to distances in meters from the center line
		x = xIntersect - xHand;
		y = yIntersect - yHand;

		%take the distances from center and convert to a unit vector,
		%then multiply by the distance to where the forces start
		%this gives us a clean number to use when calculating wall force.
		x = (x / sqrt(x^2 + y^2)) * distIntoWall;
		y = (y / sqrt(x^2 + y^2)) * distIntoWall;
	end

	%we don't want to just shut off the forces, we need to ramp them down
	%somewhat. This finds out how far into the wall we are and allows us
	%to ramp down the forces over the last 25% of the wll.
	forceRampDownZoneSizePercent = 0.75; %start ramping down the forces in the last 25% of the wall
	forceMaxEndLocInWallM = forceRampDownZoneSizePercent * wallWidthM;
	distanceIntoWall = distToLine - channelWidthM;
	scaleWallForce = 1; %assume we can run at full calculated wall force

	if distanceIntoWall > forceMaxEndLocInWallM   %we are in the ramp down zone
		distIntoRampDownZone = distanceIntoWall - forceMaxEndLocInWallM;
		rampDownZoneWidth = wallWidthM  - forceMaxEndLocInWallM;
		scaleWallForce = (rampDownZoneWidth - distIntoRampDownZone) / rampDownZoneWidth;
	end

	%within the first 1.5 seconds of the trial we don't wan to jar anyone
	%this ramps the forces up slowly so you get a gentle nudge into
	%the force channel, not a violent jerk.
	timeDelta = clockCycle - forceEnableTime;
	timeScaling = 1;
	if (timeDelta < 1500)
		timeScaling = timeDelta / 1500.0;
	end

	%the final forces will be wall force + viscous.
	forces(addIdx + 1) = (wallStiffness * scaleWallForce * timeScaling * x) + viscosityX;
	forces(addIdx + 2) = (wallStiffness * scaleWallForce  * timeScaling * y) + viscosityY;

	lastHandPosition(1) = xHand;
	lastHandPosition(2) = yHand;
end

function bIntersect = doLinesIntersect(Ap1, Ap2, Bp1, Bp2)
    %This method for finding out if 2 lines segements intersect comes from:
    %http://stackoverflow.com/questions/563198/how-do-you-detect-where-two-line-segments-intersect
   	e = Ap2-Ap1;
    f = Bp2-Bp1;
    p = [-e(2) e(1)];
    h = dot((Ap1 - Bp1), p) / dot (f, p);
    
    if h >=0 && h <= 1
        bIntersect = 1;
    else
        bIntersect = 0;
    end
end
